simulink model "Speedgoat_V4"  (R2023b)
settings: Solver=FixedStepDiscrete  StartTime=0.0  StopTime=inf  FixedStep=0.001  RelTol=1e-3  EnableMultiTasking=on
model workspace (MAT data in the model file):
  Test = 10000000
undefined symbols (not defined in the file): IO397
libraries: speedgoatlib_fpga_dio x2, speedgoatlib_fpga_analog_io x1, speedgoatlib_fpga x1
(part 2 of 2)

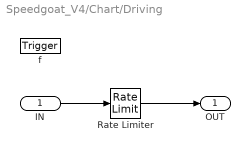
== system Speedgoat_V4/Chart/Driving ==
  IN : Inport  OutMin=[1]  OutMax=[4]  OutDataTypeStr=double  PortDimensions=1
  f : TriggerPort  TriggerType=function-call  VariantControl=(inherit)  SampleTimeType=periodic  SampleTime=0.001
      settings: CopyFcn=Stateflow.SLINSF.SimulinkMan.removeBlockPreDeleteFcn  PreDeleteFcn=Stateflow.SLINSF.SimulinkMan.unsafePredeleteFcn
  Rate Limiter : RateLimiter  RisingSlewLimit=0.01  FallingSlewLimit=-0.01  SampleTimeMode=inherited  InitialCondition=1
  OUT : Outport  OutMin=[1]  OutMax=[4]  OutputWhenDisabled=reset  InitialOutput=[1]
  wires:
  Rate Limiter/1 -> OUT/1
  IN/1 -> Rate Limiter/1

== stateflow chart Speedgoat_V4/Chart ==
  state OUT = Driving(IN) [function]
  state Distance
    du: speed_out = distance_in;
    du: Driving(distance_in);
    du: break_out = 1;
    du: direction_out = 5;
    du: cruise_out = 5;
  state IDLE
    du: speed_out = 1;
    du: Driving(1);
    du: break_out = 5;
    du: direction_out = 5;
    du: cruise_out = 5;
  state Drive
    du: speed_out = Driving(speed_in);
    du: break_out = 1;
    du: direction_out = 5;
    du: cruise_out = 5;
  state Stop
    du: speed_out = Driving(1);
    du: break_out = 1;
    du: direction_out = 5;
    du: cruise_out = 5;
  Distance -> IDLE [order 2] : [[emergency_stop_in == 1]]
  Distance -> IDLE [order 1] : [speed_out == 1]
  (default) -> IDLE
  Drive -> IDLE [order 1] : [[emergency_stop_in == 1]]
  IDLE -> Drive : [start_in == 1]
  Drive -> Distance [order 3] : [distance_in < 3.5]
  Drive -> Stop [order 2] : [stop_in == 1]
  Stop -> IDLE : [speed_out == 1]
  Distance -> Stop [order 3] : [stop_in == 1]
  data: IN function_input double size=1; OUT function_output; speed_out output; speed_in input; distance_in input; start_in input; stop_in input; break_out output; emergency_stop_in input; direction_out output; cruise_out output
